simulink model "Joint_space"  (R2023a)
settings: Solver=VariableStepAuto  StartTime=0.0  StopTime=10  RelTol=1e-3
undefined symbols (not defined in the file or in its folder): smiData, smiData1, X, Y, Z
libraries: sm_lib x261, nesl_utility x30, simulink_extras x8
(part 6 of 6)

== matlab function Joint_space/MATLAB Function2 ==
  data: q output; Tf input; t input; T output; check output
function [q,T,check]  = tasktraj(Tf,t)
    q0_traj1 = [0 ;0;0;0 ];
    qf_traj1 = [26;-26;-3;49 ];
    q0_traj2 = [26 ;-26;-3;49 ];
    qf_traj2 = [59 ;-28;-12;84 ];
    q0_traj3 = [59 ;-28;-12;84 ];
    qf_traj3 = [139 ;-29;-20;115 ];
    q0_traj4 = [139 ;-29;-20;115 ];
    qf_traj4 = [139 ;0;-45;40 ];
    q0_traj5 = [139 ;0;-45;40 ];
    qf_traj5 = [0 ;0;0;0 ];
  
    Tf1 = (Tf/5);
    Tf2= 2*(Tf/5);
    Tf3= 3*(Tf/5);
    Tf4= 4*(Tf/5);
    check =0;
    %Task_Space = [];
    if(t<=Tf1)
    q0_traj =q0_traj1;
    qf_traj =qf_traj1;
    T =t;
    check =1;
    elseif Tf1<t && t<=Tf2
    q0_traj =q0_traj2;
    qf_traj =qf_traj2;
    T = t -Tf1;
    check =2;
    elseif Tf2<t && t<=Tf3
    q0_traj =q0_traj3;
    qf_traj =qf_traj3;
    T = t -Tf2;
    check =3;
    elseif  Tf3<t && t<=Tf4
    q0_traj =q0_traj4;
    qf_traj =qf_traj4;
    T = t -Tf3;
    check =4;
    else
    q0_traj =q0_traj5;
    qf_traj =qf_traj5;
    T = t -Tf4;
    check =5;
    end

    

    c11 = (qf_traj(1)-q0_traj(1))/Tf1;
    c12 = (qf_traj(2)-q0_traj(2))/Tf1;
    c13 = (qf_traj(3)-q0_traj(3))/Tf1;
    c14 = (qf_traj(4)-q0_traj(4))/Tf1;
    q0 = q0_traj;
    q1 = q0(1) + c11*T;
    q2 = q0(2) + c12*T;
    q3 = q0(3) + c13*T;
    q4 = q0(4) + c14*T;
    
    q=[-q1;q2;-q3;q4];

== matlab function Joint_space/MATLAB Function1 ==
  data: X0 input; out1 output; Xf input; x_lift input; Tf input; t input; out2 output
function [out1,out2] = tasktraj(X0, Xf,x_lift, Tf, t)

x0=X0(1);
y0=X0(2);
z0=X0(3);
xf=Xf(1);
yf=Xf(2);
zf=Xf(3);
Tf1 = (Tf/4);
Tf2= 2*(Tf/4);
Tf3= 3*(Tf/4);
%Task_Space = [];
if(t<Tf1)
x = x0 + ((xf-x0)/Tf1)*t;
y = y0 ;
z = z0 ;
else
    if t<Tf2
    x =Xf(1);
    z=z0;
    y = y0 + ((yf-y0)/Tf1)*(t-Tf1);
    else 
        if t<Tf3
            z = z0 + ((zf-z0)/Tf1)*(t-Tf2);
            x =Xf(1);
            y=Xf(2);
        
        else
            x = xf + ((x_lift-xf)/Tf1)*(t-Tf3);
            y =Xf(2);
            z =Xf(3);
            
        end    
    end
end
out1=[x;y;z];
out2=[x+0.006;y;z];

== matlab function Joint_space/MATLAB Function3 ==
  data: q input; X output
function X = arm_forward_kinematics(q)
q1 = q(1);
q2 = q(2);
q3 = q(3);
q4 = q(4);
l1 = 0.02888;
l2 = 0.02659;
l3 = 0.1224;
l4 = 0.15;

X = [l4*cos((pi*q1)/180)*sin((pi*(q2-90))/180)*sin((pi*(q4-90))/180)-l4*cos((pi*(q4-90))/180)*(sin((pi*q1)/180)*sin((pi*(q3-90))/180)-cos((pi*q1)/180)*cos((pi*(q2-90))/180)*cos((pi*(q3-90))/180))-cos((pi*q1)/180)*sin((pi*(q2-90))/180)*(l2+l3);
    l4*cos((pi*(q4-90))/180)*(cos((pi*q1)/180)*sin((pi*(q3-90))/180)+sin((pi*q1)/180)*cos((pi*(q2-90))/180)*cos((pi*(q3-90))/180))-sin((pi*q1)/180)*sin((pi*(q2-90))/180)*(l2+l3)+l4*sin((pi*q1)/180)*sin((pi*(q2-90))/180)*sin((pi*(q4-90))/180);
    l4*cos((pi*(q2-90))/180)*sin((pi*(q4-90))/180)-cos((pi*(q2-90))/180)*(l2+l3)-l1-l4*cos((pi*(q3-90))/180)*cos((pi*(q4-90))/180)*sin((pi*(q2-90))/180)];
      
x = X(1,1);
y = X(2,1);
z = X(3,1);
X = [x;y;z]
